simulink model "solor_model_exp"  (R2020a)
settings: Solver=ode45  StartTime=0.0  StopTime=10.0  RelTol=1e-3  EnableMultiTasking=on
InitFcn:
  | load pr
StartFcn:
  | load pr
values from neighbouring files (symbols this model uses):
  opt = 75    [pr.mat]    (also in solor_irra_var.m = 30; solor_temp_var.m = temp(i))
  srad = 500    [pr.mat]    (also in solor_irra_var.m = srd(i); solor_temp_var.m)
libraries: simulink x2, powerlib x1
settings Model: Creator=Rajora  LastModifiedBy=shrad
settings DataIOCC: LimitDataPoints=on  SaveFormat=Array  SignalLoggingSaveFormat=ModelDataLogs  ReturnWorkspaceOutputs=off
settings OptimizationCC: ExpressionDepthLimit=2147483647  LifeSpan=inf
settings DebuggingCC: UnderspecifiedInitializationDetection=Classic  MergeDetectMultiDrivingBlocksExec=none  SolverPrmCheckMsg=warning  FcnCallInpInsideContextMsg=warning  StateNameClashWarn=warning  SFUnexpectedBacktrackingDiag=warning  SFNoUnconditionalDefaultTransitionDiag=warning  SFExecutionAtInitializationDiag=none  ArithmeticOperatorsInVariantConditions=warning
settings HardwareCC: ProdBitPerPointer=32  ProdBitPerSizeT=32  ProdBitPerPtrDiffT=32  ProdLargestAtomicFloat=None  ProdIntDivRoundTo=Undefined  ProdEndianess=Unspecified  ProdWordSize=32  ProdHWDeviceType=32-bit Generic
settings ModelReferenceCC: PropagateSignalLabelsOutOfModel=off
settings SFSimCC: SimUseLocalCustomCode=off  CustomCodeUndefinedFunction=UseInterfaceOnly
settings RTWCC: RTWUseLocalCustomCode=off
settings CodeAppCC: StateflowObjectComments=on
settings GRTTargetCC: TargetLangStandard=C89/C90 (ANSI)
settings ConfigComp: CovMetricSettings=dw  CovHtmlReporting=on  CovSaveCumulativeToWorkspaceVar=on  CovSaveSingleToWorkspaceVar=on  CovExternalEMLEnable=off
settings SimscapeCC: SimscapeNormalizeSystem=off
settings ConfigurationSet: Description=SimMechanics 2G

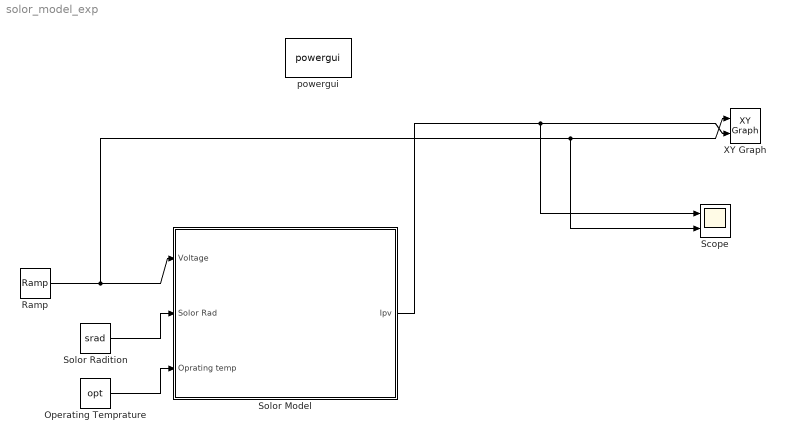
== system solor_model_exp ==
  Operating Temprature : Constant  Value=opt
  Ramp : simulink/Sources/Ramp  slope=3  start=0  InitialOutput=0
  Scope : Scope  NumInputPorts=2
  Solor Model : Subsystem
  Solor Radition : Constant  Value=srad
  XY Graph : simulink/Sinks/XY Graph  xmin=-1  xmax=22  ymin=-1  ymax=10  st=-1
  powergui : powerlib/powergui  Priority=1  SimulationMode=Discrete  SampleTime=1e-6  frequency=60  Iterations=50  frequencyindice=0  Pbase=100e6  ErrMax=1e-4  UnitsV=kV  UnitsW=MW  buscounter=0  FunctionMessages=off  echomessages=off  EnableUseOfTLC=off  CurrentSourceSwitches=off  DisableSnubberDevices=off  DisableRonSwitches=off  DisableVfSwitches=off  DisplayEquations=off  AutomaticDiscreteSolvers=off  SolverType=Tustin  Interpol=off  ExternalGateDelay=off  methode=off  Ts=0  x0status=blocks  SPID=off  SwTol=0  HookPort=off  NonlinearTolerance=1e-4  nMaxIteration=100  ContinueOnMaxIteration=off  RestoreLinks=warning  ResistiveCurrentMeasurement=off  Frange=[0:2:500]  Ylog=off  Xlog=on  ShowGrid=off  save=off  variable=ZData  structure=0  ZoomFFT=off  StartTime=0.0  cycles=1  DisplayStyle=1  fundamental=60  FreqAxis=off  MaxFrequency=1000  frequencyindicesteady=1  RmsSteady=1  display=off
  wires:
  Operating Temprature/1 -> Solor Model/3(Oprating temp)
  Solor Radition/1 -> Solor Model/2(Solor Rad)
  Solor Model/1(Ipv) -> XY Graph/2, Scope/1
  Ramp/1 -> Solor Model/1(Voltage), XY Graph/1, Scope/2

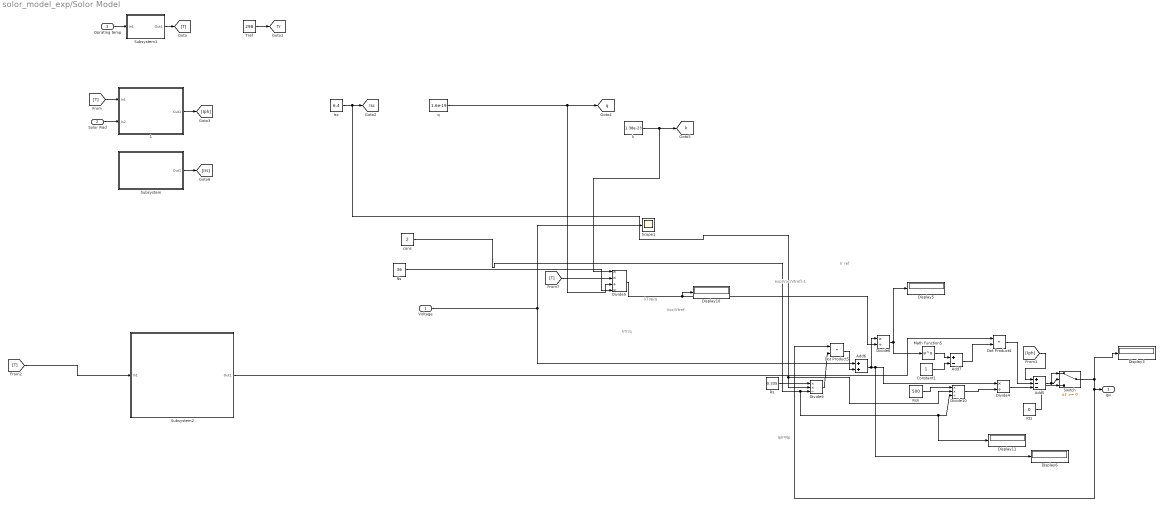
== system solor_model_exp/Solor Model ==
  note: kTop/q
  note: Iph*Np
  note: kTr/q
  note: Voc/Vtref
  note: exp(Voc/Vtref)-1
  note: Ir ref
  Voltage : Inport
  Solor Rad : Inport  Port=2
  Oprating temp : Inport  Port=3
  1 : Subsystem
  Add5 : Sum  Inputs=+--
  Add6 : Sum
  Add7 : Sum  Inputs=+-
  Constant1 : Constant
  Display{3,5..6,10..11} (5 alike) : Display
  Divide10 : Product  Inputs=**/
  Divide4 : Product  Inputs=*/
  Divide5 : Product  Inputs=**/*
  Divide6 : Product  Inputs=*/
  Divide9 : Product  Inputs=**/
  Dot Product4 : DotProduct  InputSameDT=on  OutDataTypeStr=Inherit: Inherit via internal rule
  Dot Product5 : DotProduct  InputSameDT=on  OutDataTypeStr=Inherit: Inherit via internal rule
  Isc : Constant  Value=6.4
  Kt1 : Constant  Value=0
  Math Function5 : Math  SignedPower=on  SaturateOnIntegerOverflow=on
  Ns : Constant  Value=36
  Rs : Constant  Value=0.335
  Rsh : Constant  Value=500
  Scope1 : Scope
  Subsystem : Subsystem
  Subsystem1 : Subsystem
  Subsystem2 : Subsystem
  Switch : Switch
  Tref : Constant  Value=298
  cons : Constant  Value=2
  k : Constant  Value=1.38e-23
  q : Constant  Value=1.6e-19
  Ipv : Outport
  tag scope: Isc=global, Tr=global, k=global, q=global
  wires:
  Isc/1 -> Divide9/2, Divide10/2, [Isc]
  Voltage/1 -> Add6/1, Scope1/1
  Dot Product4/1 -> Add5/2
  Dot Product5/1 -> Add6/2
  Add6/1 -> Divide4/1, Display6/1, Divide6/1
  Divide4/1 -> Add5/3
  q/1 -> [q], Divide5/3
  Divide5/1 -> Divide6/2, Display10/1
  Constant1/1 -> Add7/2
  Add7/1 -> Dot Product4/2
  Math Function5/1 -> Add7/1
  Divide6/1 -> Math Function5/1, Display5/1
  Add5/1 -> Switch/2, Switch/1
  Switch/1 -> Dot Product5/1, Ipv/1, Display3/1
  Tref/1 -> [Tr]
  Ns/1 -> Divide5/4
  cons/1 -> Divide9/3, Divide10/3, Display11/1
  Rs/1 -> Divide9/1
  Divide9/1 -> Dot Product5/2
  Rsh/1 -> Divide10/1
  Divide10/1 -> Divide4/2
  k/1 -> [k], Divide5/1
  Kt1/1 -> Switch/3
  1/1(Out1) -> [Iph]
  [T] -> 1/1(In1)
  Solor Rad/1 -> 1/2(In2)
  [Iph] -> Add5/1
  Subsystem/1(Out1) -> [Irs]
  Subsystem1/1(Out1) -> [T]
  Oprating temp/1 -> Subsystem1/1(In1)
  [T] -> Divide5/2
  [T] -> Subsystem2/1(In1)
  Subsystem2/1(Out1) -> Dot Product4/1

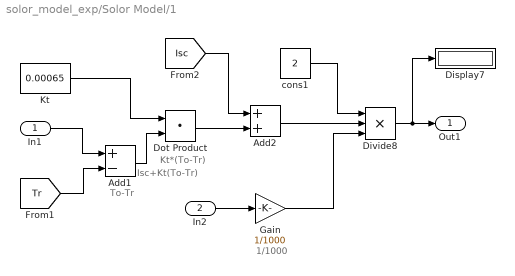
== system solor_model_exp/Solor Model/1 ==
  note: To-Tr
  note: Kt*(To-Tr)
  note: Isc+Kt(To-Tr)
  note: 1/1000
  In1 : Inport
  In2 : Inport  Port=2
  Add1 : Sum  Inputs=+-
  Add2 : Sum
  Display7 : Display
  Divide8 : Product  Inputs=***
  Dot Product : DotProduct  InputSameDT=on  OutDataTypeStr=Inherit: Inherit via internal rule
  Gain : Gain  Gain=1/1000
  Kt : Constant  Value=0.00065
  cons1 : Constant  Value=2
  Out1 : Outport
  wires:
  Dot Product/1 -> Add2/2
  cons1/1 -> Divide8/1
  [Isc] -> Add2/1
  [Tr] -> Add1/2
  Kt/1 -> Dot Product/1
  Divide8/1 -> Display7/1, Out1/1
  Add2/1 -> Divide8/2
  Gain/1 -> Divide8/3
  Add1/1 -> Dot Product/2
  In2/1 -> Gain/1
  In1/1 -> Add1/1

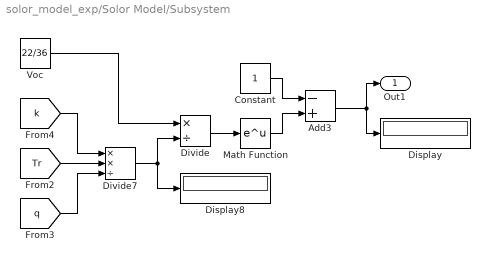
== system solor_model_exp/Solor Model/Subsystem ==
  Add3 : Sum  Inputs=-+
  Constant : Constant
  Display : Display
  Display8 : Display
  Divide : Product  Inputs=*/
  Divide7 : Product  Inputs=**/
  Math Function : Math  SignedPower=on  SaturateOnIntegerOverflow=on
  Voc : Constant  Value=22/36
  Out1 : Outport
  wires:
  [k] -> Divide7/1
  Voc/1 -> Divide/1
  [q] -> Divide7/3
  Add3/1 -> Out1/1, Display/1
  [Tr] -> Divide7/2
  Divide/1 -> Math Function/1
  Math Function/1 -> Add3/2
  Divide7/1 -> Divide/2, Display8/1
  Constant/1 -> Add3/1

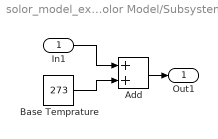
== system solor_model_exp/Solor Model/Subsystem1 ==
  In1 : Inport
  Add : Sum
  Base Temprature : Constant  Value=273
  Out1 : Outport
  wires:
  Add/1 -> Out1/1
  Base Temprature/1 -> Add/2
  In1/1 -> Add/1

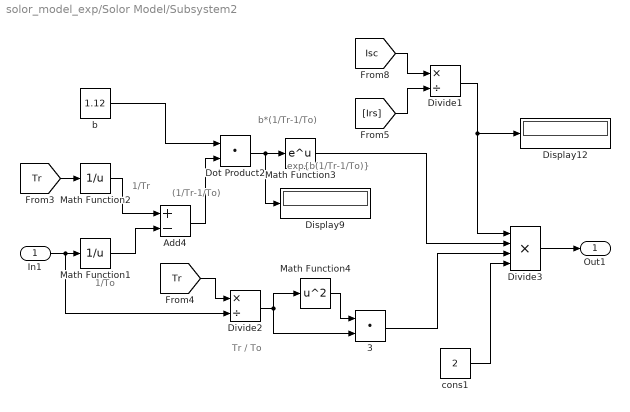
== system solor_model_exp/Solor Model/Subsystem2 ==
  note: Tr / To
  note: 1/Tr
  note: 1/To
  note: (1/Tr-1/To)
  note: b*(1/Tr-1/To)
  note: exp{b(1/Tr-1/To)}
  In1 : Inport
  3 : DotProduct  InputSameDT=on  OutDataTypeStr=Inherit: Inherit via internal rule
  Add4 : Sum  Inputs=+-
  Display12 : Display
  Display9 : Display
  Divide1 : Product  Inputs=*/
  Divide2 : Product  Inputs=*/
  Divide3 : Product  Inputs=****
  Dot Product2 : DotProduct  InputSameDT=on  OutDataTypeStr=Inherit: Inherit via internal rule
  Math Function1 : Math  Operator=reciprocal  SignedPower=on  SaturateOnIntegerOverflow=on
  Math Function2 : Math  Operator=reciprocal  SignedPower=on  SaturateOnIntegerOverflow=on
  Math Function3 : Math  SignedPower=on  SaturateOnIntegerOverflow=on
  Math Function4 : Math  Operator=square  SignedPower=on  SaturateOnIntegerOverflow=on
  b : Constant  Value=1.12
  cons1 : Constant  Value=2
  Out1 : Outport
  wires:
  [Tr] -> Math Function2/1
  Math Function4/1 -> 3/1
  Divide2/1 -> 3/2, Math Function4/1
  3/1 -> Divide3/3
  Math Function3/1 -> Divide3/2
  In1/1 -> Divide2/2, Math Function1/1
  b/1 -> Dot Product2/1
  Math Function2/1 -> Add4/1
  Add4/1 -> Dot Product2/2
  Divide1/1 -> Display12/1, Divide3/1
  Math Function1/1 -> Add4/2
  Dot Product2/1 -> Math Function3/1, Display9/1
  [Tr] -> Divide2/1
  [Isc] -> Divide1/1
  cons1/1 -> Divide3/4
  [Irs] -> Divide1/2
  Divide3/1 -> Out1/1
